simulink model "TugLibrary"  (R2019a)
settings: Solver=VariableStepAuto  StartTime=0.0  StopTime=10.0  RelTol=1e-3
libraries: arduinolib x4
settings Model: Creator=Asus  LastModifiedBy=Asus

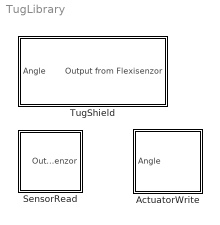
== system TugLibrary ==
  ActuatorWrite : Subsystem  Description=Sets angle of servo arm. Servo is part of TugShield board, which bend flexi sensor. Expects input in the range of 0-180 degrees.
      mask help: The ActuatorWrite function block is used to set the angle of the servo arm on TugShield board. Expects input in the range of 0-180°.
      mask Display: image('Obr_vstup.jpg');
  "SensorRead " : Subsystem  mask{OutRadio=ADC levels, Ts=0.005, CalType=Manual, MinVal=0, MaxVal=675}
      mask prompts: OutRadio "Output type"; Ts "Sampling period (s)"; CalType "Calibration values"; MinVal "Minimum"; MaxVal "Maximum"
      mask help: The SensorRead function block reads the value from the flexi sensor located on pine A0.
      mask init:
      | if CalType==1    
      |     set_param(gcb,'MinVal',num2str(0));
      |     set_param(gcb,'MaxVal',num2str(675));    
      | end
      mask TypeOptions OutRadio: ADC levels | Percent (%)
      mask Callback OutRadio:
      | CurrentBlock = gcb;
      | Output = get_param(CurrentBlock,'OutRadio');
      | Calib = get_param(CurrentBlock,'CalType');
      | Menu = Simulink.Mask.get(CurrentBlock);
      | CalibOpt = Menu.getParameter('CalType');
      | MinOpt = Menu.getParameter('MinVal');
      | MaxOpt = Menu.getParameter('MaxVal');
      | 
      | if strcmp(Output,'ADC levels')
      | CalibOpt.Enabled='off';
      | MinOpt.Enabled='off';
      | MaxOpt.Enabled='off';
      | elseif strcmp(Calib,'Manual')
      | CalibOpt.Enabled='on';
      | MinOpt.Enabled='on';
      | MaxOpt.Enabled='on';
      | else
      | CalibOpt.Enabled='on';
      | MinOpt.Enabled='off';
      | MaxOpt.Enabled='off';
      | end
      mask TypeOptions CalType: Default value (recommended) | Manual
      mask Callback CalType:
      | CurrentBlock = gcbh;
      | Output = get_param(CurrentBlock,'OutRadio');
      | Calib = get_param(CurrentBlock,'CalType');
      | Menu = Simulink.Mask.get(CurrentBlock);
      | MinOpt = Menu.getParameter('MinVal');
      | MaxOpt = Menu.getParameter('MaxVal');
      | 
      | if strcmp(Output,'ADC levels')
      | MinOpt.Enabled='off';
      | MaxOpt.Enabled='off';
      | elseif strcmp(Calib,'Manual')
      | MinOpt.Enabled='on';
      | MaxOpt.Enabled='on';
      | else
      | MinOpt.Enabled='off';
      | MaxOpt.Enabled='off';
      | end
      mask DialogControl DescGroupVar Prompt: TugShield Flexi Sensor
      mask DialogControl DescTextVar Prompt: The SensorRead function block reads the value from the flexi sensor located on pine A0.
      mask Display: image('Obr_vystup.png');
  TugShield : Subsystem  mask{OutRadio=ADC levels, Ts=0.005, CalType=Default settings (recommended), MinVal=0, MaxVal=675}
      mask prompts: OutRadio "Output type"; Ts "Sampling period (s)"; CalType "Calibration valueas"; MinVal "Minimal"; MaxVal "Maximal"
      mask help:
      | TugShield block connects two block - SensorRead and ActuatorWrite.
      | Input signal is written to the ActuatorWrite block, which sets angle of servo arm and then the output signal from flexi sensor is read by ActuarotWrite block.
      mask init:
      | if CalType==1    
      |     set_param(gcb,'MinVal',num2str(0));
      |     set_param(gcb,'MaxVal',num2str(675));    
      | end
      mask TypeOptions OutRadio: ADC levels | Percent (%)
      mask Callback OutRadio:
      | CurrentBlock = gcb;
      | Output = get_param(CurrentBlock,'OutRadio');
      | Calib = get_param(CurrentBlock,'CalType');
      | Menu = Simulink.Mask.get(CurrentBlock);
      | CalibOpt = Menu.getParameter('CalType');
      | MinOpt = Menu.getParameter('MinVal');
      | MaxOpt = Menu.getParameter('MaxVal');
      | 
      | if strcmp(Output,'ADC levels')
      | CalibOpt.Enabled='off';
      | MinOpt.Enabled='off';
      | MaxOpt.Enabled='off';
      | elseif strcmp(Calib,'Manual')
      | CalibOpt.Enabled='on';
      | MinOpt.Enabled='on';
      | MaxOpt.Enabled='on';
      | else
      | CalibOpt.Enabled='on';
      | MinOpt.Enabled='off';
      | MaxOpt.Enabled='off';
      | end
      mask TypeOptions CalType: Default settings (recommended) | Manual
      mask Callback CalType:
      | CurrentBlock = gcbh;
      | Output = get_param(CurrentBlock,'OutRadio');
      | Calib = get_param(CurrentBlock,'CalType');
      | Menu = Simulink.Mask.get(CurrentBlock);
      | MinOpt = Menu.getParameter('MinVal');
      | MaxOpt = Menu.getParameter('MaxVal');
      | 
      | if strcmp(Output,'ADC levels')
      | MinOpt.Enabled='off';
      | MaxOpt.Enabled='off';
      | elseif strcmp(Calib,'Manual')
      | MinOpt.Enabled='on';
      | MaxOpt.Enabled='on';
      | else
      | MinOpt.Enabled='off';
      | MaxOpt.Enabled='off';
      | end
      mask DialogControl DescGroupVar Prompt: TugShield
      mask DialogControl DescTextVar Prompt: TugShield block connects two block - SensorRead and ActuatorWrite. Input signal is written to the ActuatorWrite block, which sets angle of servo arm and then the output signal from flexi sensor is read by ActuarotWrite block.
      mask Display: image('Obr_vstupvystup.png');

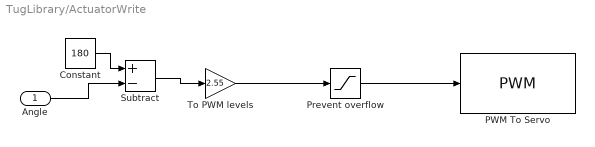
== system TugLibrary/ActuatorWrite ==
  Angle : Inport
  Constant : Constant  Value=180
  PWM To Servo : arduinolib/PWM  pinNumber=10  EnableInputFrequency=off  InitialFrequency=2000  InitialDutyCycle=0  NotificationType=None  blockPlatform=arduino
  Prevent overflow : Saturate  UpperLimit=255  LowerLimit=0
  Subtract : Sum  Inputs=+-
  To PWM levels : Gain  Gain=2.55
  wires:
  Constant/1 -> Subtract/1
  To PWM levels/1 -> Prevent overflow/1
  Prevent overflow/1 -> PWM To Servo/1
  Angle/1 -> Subtract/2
  Subtract/1 -> To PWM levels/1

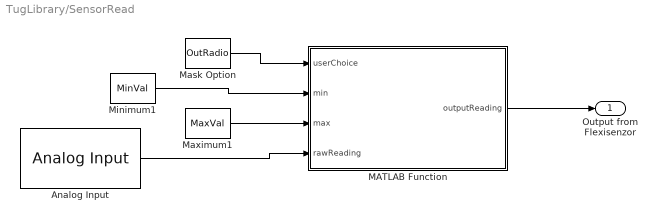
== system TugLibrary/SensorRead  ==
  Analog Input : arduinolib/Analog Input  pinNumber=0  ReadResultsOnly=off  ConversionTriggerSource=Software  ExternalTriggerType=uint32(0)  OutputDataType=uint16  EnableConversionCompleteNotify=off  EnableOuputStatus=off  SampleTime=Ts  blockPlatform=arduino
  MATLAB Function : MATLAB Function  TreatAsAtomicUnit=on
  Mask Option : Constant  Value=OutRadio  SampleTime=Ts
  Maximum1 : Constant  Value=MaxVal  SampleTime=Ts
  Minimum1 : Constant  Value=MinVal  SampleTime=Ts
  Output from Flexisenzor : Outport
  wires:
  Mask Option/1 -> MATLAB Function/1(userChoice)
  Minimum1/1 -> MATLAB Function/2(min)
  Maximum1/1 -> MATLAB Function/3(max)
  Analog Input/1 -> MATLAB Function/4(rawReading)
  MATLAB Function/1(outputReading) -> Output from Flexisenzor/1

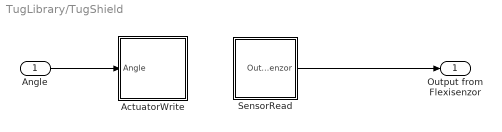
== system TugLibrary/TugShield ==
  Angle : Inport
  ActuatorWrite : Subsystem  Description=Sets angle of servo arm. Servo is part of TugShield board, which bend flexi sensor. Expects input in the range of 0-180 degrees.
      mask help: The ActuatorWrite function block is used to set the angle of the servo arm on TugShield board. Expects input in the range of 0-180°.
      mask Display: image('Obr_vstup.jpg');
  "SensorRead " : Subsystem  mask{OutRadio=Percent (%), Ts=0.005, CalType=Default value (recommended), MinVal=0, MaxVal=675}
      mask prompts: OutRadio "Output type"; Ts "Sampling period (s)"; CalType "Calibration values"; MinVal "Minimum"; MaxVal "Maximum"
      mask help: The SensorRead function block reads the value from the flexi sensor located on pine A0.
      mask init:
      | if CalType==1    
      |     set_param(gcb,'MinVal',num2str(0));
      |     set_param(gcb,'MaxVal',num2str(675));    
      | end
      mask TypeOptions OutRadio: ADC levels | Percent (%)
      mask TypeOptions CalType: Default value (recommended) | Manual
      mask DialogControl DescGroupVar Prompt: TugShield Flexi Sensor
      mask DialogControl DescTextVar Prompt: The SensorRead function block reads the value from the flexi sensor located on pine A0.
      mask Display: image('Obr_vystup.png');
  Output from Flexisenzor : Outport
  wires:
  "SensorRead "/1(Output from Flexisenzor) -> Output from Flexisenzor/1
  Angle/1 -> ActuatorWrite/1(Angle)

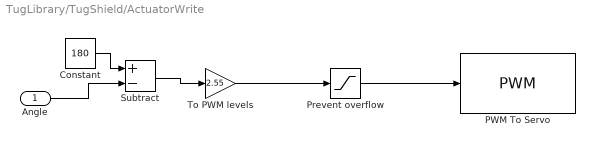
== system TugLibrary/TugShield/ActuatorWrite ==
  Angle : Inport
  Constant : Constant  Value=180
  PWM To Servo : arduinolib/PWM  pinNumber=10  EnableInputFrequency=off  InitialFrequency=2000  InitialDutyCycle=0  NotificationType=None  blockPlatform=arduino
  Prevent overflow : Saturate  UpperLimit=255  LowerLimit=0
  Subtract : Sum  Inputs=+-
  To PWM levels : Gain  Gain=2.55
  wires:
  Constant/1 -> Subtract/1
  To PWM levels/1 -> Prevent overflow/1
  Prevent overflow/1 -> PWM To Servo/1
  Angle/1 -> Subtract/2
  Subtract/1 -> To PWM levels/1

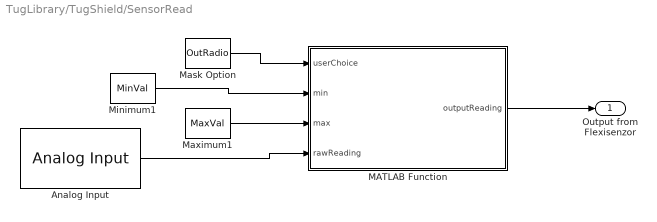
== system TugLibrary/TugShield/SensorRead  ==
  Analog Input : arduinolib/Analog Input  pinNumber=0  ReadResultsOnly=off  ConversionTriggerSource=Software  ExternalTriggerType=uint32(0)  OutputDataType=uint16  EnableConversionCompleteNotify=off  EnableOuputStatus=off  SampleTime=Ts  blockPlatform=arduino
  MATLAB Function : MATLAB Function  TreatAsAtomicUnit=on
  Mask Option : Constant  Value=OutRadio  SampleTime=Ts
  Maximum1 : Constant  Value=MaxVal  SampleTime=Ts
  Minimum1 : Constant  Value=MinVal  SampleTime=Ts
  Output from Flexisenzor : Outport
  wires:
  Mask Option/1 -> MATLAB Function/1(userChoice)
  Minimum1/1 -> MATLAB Function/2(min)
  Maximum1/1 -> MATLAB Function/3(max)
  Analog Input/1 -> MATLAB Function/4(rawReading)
  MATLAB Function/1(outputReading) -> Output from Flexisenzor/1

== matlab function TugLibrary/TugShield/SensorRead /MATLAB Function ==
  data: userChoice input; outputReading output; min input; max input; rawReading input
%     Matlab function for Sensor Read block functionality.
%
%     This code is part of the AutomationShield hardware and software
%     ecosystem. Visit http://www.automationshield.com for more
%     details. This code is licensed under a Creative Commons
%     Attribution-NonCommercial 4.0 International License.
%
%     Created by Eva Vargová.
%     Last update: 3.3.2021.

function outputReading = fcn(userChoice, min, max, rawReading)
    if userChoice == 1
        outputReading = rawReading;
    else
        outputReading = constrain(map(rawReading, max, min, 0, 100), 0, 100);
    end
end

== matlab function TugLibrary/SensorRead /MATLAB Function ==
  data: userChoice input; outputReading output; min input; max input; rawReading input
%     Matlab function for Sensor Read block functionality.
%
%     This code is part of the AutomationShield hardware and software
%     ecosystem. Visit http://www.automationshield.com for more
%     details. This code is licensed under a Creative Commons
%     Attribution-NonCommercial 4.0 International License.
%
%     Created by Eva Vargová.
%     Last update: 3.3.2021.

function outputReading = fcn(userChoice, min, max, rawReading)
    if userChoice == 1
        outputReading = rawReading;
    else
        outputReading = constrain(map(rawReading, max, min, 0, 100), 0, 100);
    end
end
